simulink model "ASMCDUNG"  (R2022b)
settings: Solver=ode45  StartTime=0.0  StopTime=30  FixedStep=0.05  RelTol=1e-3
libraries: slpidlib x2
settings Model: Creator=vudin  LastModifiedBy=vudin
settings SolverCC: AlgebraicLoopSolver=TrustRegion
settings DataIOCC: ReturnWorkspaceOutputs=off
settings DebuggingCC: UnconnectedInputMsg=warning  UnconnectedOutputMsg=warning  UnconnectedLineMsg=warning  SFMachineParentedDataDiag=warning  ArithmeticOperatorsInVariantConditions=warning
settings ModelReferenceCC: EnableRefExpFcnMdlSchedulingChecks=on
settings SFSimCC: CustomCodeUndefinedFunction=UseInterfaceOnly

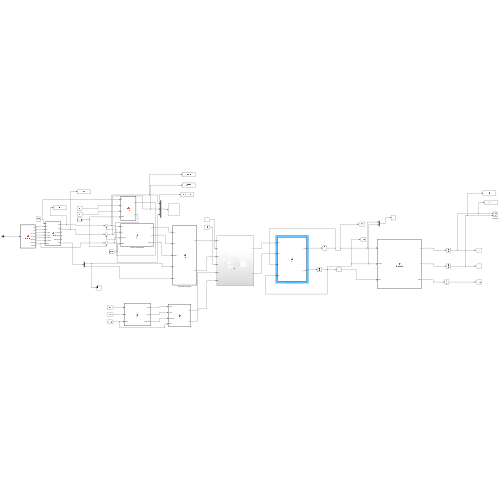
[thumbnail: Simulink's stored preview of the top-level diagram]
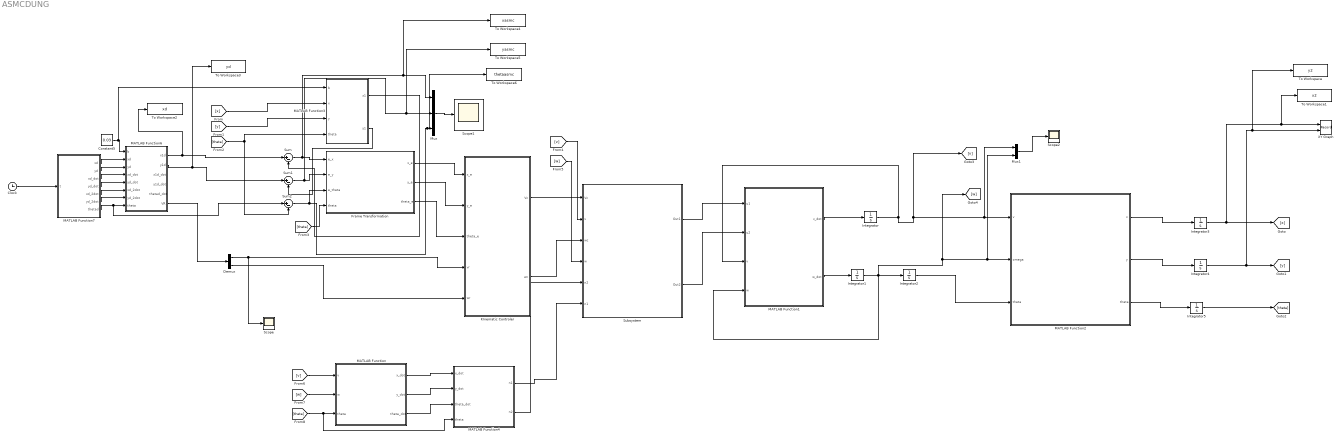
== system ASMCDUNG ==
  Clock : Clock
  Constant5 : Constant  Value=0.03
  Demux : Demux  Outputs=2
  Frame Transformation : MATLAB Function  TreatAsAtomicUnit=on
  Integrator{,1..5} (6 alike) : Integrator
  KInematic Controler : MATLAB Function  TreatAsAtomicUnit=on
  MATLAB Function : MATLAB Function  TreatAsAtomicUnit=on
  MATLAB Function1 : MATLAB Function  TreatAsAtomicUnit=on
  MATLAB Function2 : MATLAB Function  TreatAsAtomicUnit=on
  MATLAB Function3 : MATLAB Function  TreatAsAtomicUnit=on
  MATLAB Function4 : MATLAB Function  TreatAsAtomicUnit=on
  MATLAB Function6 : MATLAB Function  TreatAsAtomicUnit=on
  MATLAB Function7 : MATLAB Function  TreatAsAtomicUnit=on
  Mux : Mux  Inputs=3
  Mux1 : Mux  Inputs=2
  Scope : Scope
  Scope1 : Scope
  Scope2 : Scope
  Subsystem : Subsystem
  Sum : Sum  Inputs=|+-
  Sum1 : Sum  Inputs=|+-
  Sum2 : Sum  Inputs=|+-
  To Workspace : ToWorkspace  VariableName=y2  SampleTime=-1
  To Workspace1 : ToWorkspace  VariableName=x2  SampleTime=-1
  To Workspace2 : ToWorkspace  VariableName=xd  SaveFormat=Timeseries  SampleTime=-1
  To Workspace3 : ToWorkspace  VariableName=yd  SaveFormat=Timeseries  SampleTime=-1
  To Workspace4 : ToWorkspace  VariableName=xasmc  SaveFormat=Timeseries  SampleTime=-1
  To Workspace5 : ToWorkspace  VariableName=yasmc  SaveFormat=Timeseries  SampleTime=-1
  To Workspace6 : ToWorkspace  VariableName=thetaasmc  SaveFormat=Timeseries  SampleTime=-1
  XY Graph : Record  FileSettingsInternal="{\"entries\":[{\"content\":{\"excelSettings\":{\"content\":{},\"type\":\"Streamout.ExcelSettings\"}},\"type\":\"Streamout.FileSettingStorage\",\"uuid\":\"6435c98a-ca60-4c6a-9dec-2f97648765b9\"}],\"packageUris\":[\"http://schema.mathworks.com/mf0/streamout_blocks/R2020a\"],\"version\":\"1.0\"}"  Layout=[1 1]  SignalsInternal="{\"entries\":[{\"content\":{\"signals\":[{\"content\":{\"blockPath\":[\"ASMCDUNG/XY Graph\"],\"channel\":[],\"dimensions\":[1],\"domain\":\"ASMCDUNG/XY Graph\",\"lineColor\":\"#a2142f\",\"plots\":[1],\"port\":1,\"sid\":[\"\"],\"signalID\":19,\"signalName\":\"Integrator3\"},\"type\":\"RecordBlkView.Signal\",\"uuid\":\"5e08760f-4a30-4797-bcab-71919d67c0cf\"},{\"content\":{\"blockPath\":[\"ASMCDUNG/XY Graph\"],\"channel\":[],\"dimensions\":[1],\"domain\":\"ASMCDUNG/XY Graph\",\"lineColor\":\"#139fff\",\"plots\":[1],\"port\":2,\"sid\":[\"\"],\"signalID\":23,\"signalName\":\"Integrator4\"},\"type\":\"RecordBlkView.Signal\",\"uuid\":\"f2d516c6-4b6f-479c-badf-737930e26c05\"}]},\"type\":\"RecordBlkView.InputSignals\",\"uuid\":\"03edcad2-6278-41f4-8767-b85c0ff9a77c\"}],\"packageUris\":[\"http://schema.mathworks.com/mf0/streamout_blocks/R2020a\"],\"version\":\"1.0\"}"  VisualizationBindings="{\"xyplotplugin\":{\"info\":[{\"series\":[{\"bindingParametersList\":[{\"parameter\":\"X-Axis\",\"signalID\":19,\"signalName\":\"Integrator3\"},{\"parameter\":\"Y-Axis\",\"signalID\":23,\"signalName\":\"Integrator4\"}],\"seriesID\":10262}],\"subplotID\":1}]}}"  CompatibilityTag=XY  st=-1
  wires:
  Frame Transformation/2(y_e) -> KInematic Controler/2(y_e)
  MATLAB Function3/1(x1) -> Sum/2
  Integrator4/1 -> To Workspace/1, XY Graph/2, [y]
  [theta] -> Frame Transformation/4(theta)
  [theta] -> MATLAB Function4/4(theta), MATLAB Function/3(theta)
  MATLAB Function/2(y_dot) -> MATLAB Function4/2(y_dot)
  [w] -> MATLAB Function/2(w)
  Subsystem/2(Out2) -> MATLAB Function1/2(u2)
  [x] -> MATLAB Function3/2(x)
  Demux/2 -> KInematic Controler/5(wr)
  [v] -> MATLAB Function/1(v)
  MATLAB Function7/4(yd_dot) -> MATLAB Function6/5(yd_dot)
  Frame Transformation/1(x_e) -> KInematic Controler/1(x_e)
  [y] -> MATLAB Function3/3(y)
  Frame Transformation/3(theta_e) -> KInematic Controler/3(theta_e)
  MATLAB Function/3(theta_dot) -> MATLAB Function4/3(theta_dot)
  Sum1/1 -> To Workspace5/1, Mux/2, Frame Transformation/2(e_y)
  Sum2/1 -> To Workspace6/1, Mux/3, Frame Transformation/3(e_theta)
  MATLAB Function7/6(yd_2dot) -> MATLAB Function6/7(yd_2dot)
  Demux/1 -> Scope/1, KInematic Controler/4(vr)
  [v] -> Subsystem/2(v)
  Subsystem/1(Out1) -> MATLAB Function1/1(u1)
  MATLAB Function7/1(xd) -> MATLAB Function6/2(xd)
  MATLAB Function2/1(x) -> Integrator3/1
  Mux1/1 -> Scope2/1
  MATLAB Function7/7(thetad) -> Sum2/1, MATLAB Function6/8(theta)
  KInematic Controler/2(wc) -> Subsystem/3(wc)
  Constant5/1 -> MATLAB Function3/1(b), MATLAB Function6/1(b)
  MATLAB Function7/2(yd) -> MATLAB Function6/3(yd)
  MATLAB Function7/3(xd_dot) -> MATLAB Function6/4(xd_dot)
  MATLAB Function6/6(VR) -> Demux/1
  Sum/1 -> Frame Transformation/1(e_x), To Workspace4/1, Mux/1
  Integrator/1 -> MATLAB Function1/3(v), [v], Mux1/1, MATLAB Function2/1(v)
  MATLAB Function3/2(y1) -> Sum1/2
  Integrator5/1 -> [theta]
  [w] -> Subsystem/4(w)
  MATLAB Function4/2(n2) -> Subsystem/5(n2)
  MATLAB Function1/1(v_dot) -> Integrator/1
  MATLAB Function1/2(w_dot) -> Integrator1/1
  MATLAB Function6/1(x1d) -> To Workspace2/1, Sum/1
  MATLAB Function/1(x_dot) -> MATLAB Function4/1(x_dot)
  MATLAB Function2/2(y) -> Integrator4/1
  MATLAB Function6/2(y1d) -> To Workspace3/1, Sum1/1
  MATLAB Function2/3(theta) -> Integrator5/1
  [theta] -> Sum2/2, MATLAB Function3/4(theta)
  Integrator3/1 -> To Workspace1/1, XY Graph/1, [x]
  KInematic Controler/1(Vc) -> Subsystem/1(Vc)
  Integrator1/1 -> [w], Mux1/2, MATLAB Function2/2(omega), MATLAB Function1/4(w), Integrator2/1
  MATLAB Function4/1(n1) -> Subsystem/6(n1)
  Mux/1 -> Scope1/1
  Integrator2/1 -> MATLAB Function2/3("theta ")
  MATLAB Function7/5(xd_2dot) -> MATLAB Function6/6(xd_2dot)
  Clock/1 -> MATLAB Function7/1(t)

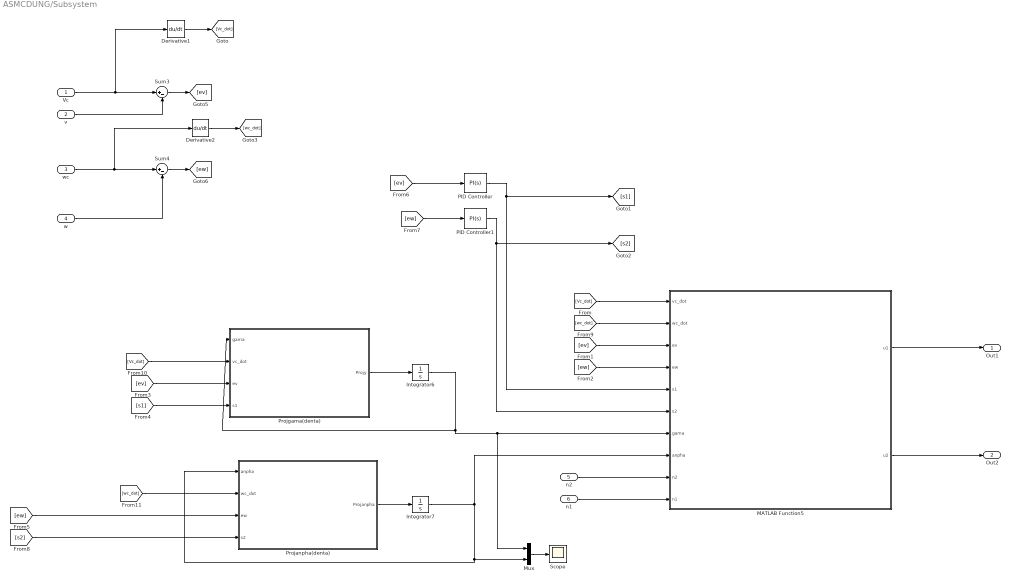
== system ASMCDUNG/Subsystem ==
  Vc : Inport
  v : Inport  Port=2
  wc : Inport  Port=3
  w : Inport  Port=4
  n2 : Inport  Port=5
  n1 : Inport  Port=6
  Derivative1 : Derivative
  Derivative2 : Derivative
  Integrator6 : Integrator
  Integrator7 : Integrator
  MATLAB Function5 : MATLAB Function  TreatAsAtomicUnit=on
  Mux : Mux  Inputs=2
  PID Controller : slpidlib/PID Controller  Controller=PI  Form=Parallel  TimeDomain=Continuous-time  UseExternalTs=off  SampleTime=-1  IntegratorMethod=Forward Euler  FilterMethod=Forward Euler  ControllerParametersSource=internal  P=3.4  I=1  UseKiTs=off  D=0  N=100  UseFilter=on  TunerSelectOption=Transfer Function Based (PID Tuner App)  InitialConditionSource=internal  InitialConditionForIntegrator=0  InitialConditionForFilter=0  DifferentiatorICPrevScaledInput=0  ExternalReset=none  TrackingMode=off  Kt=1  LimitOutput=off  SatLimitsSource=internal  UpperSaturationLimit=inf  LowerSaturationLimit=-inf  LinearizeAsGain=on  AntiWindupMode=none  Kb=1  LimitIntegrator=off  UpperIntegratorSaturationLimit=inf  LowerIntegratorSaturationLimit=-inf  POutMin=[]  POutMax=[]  IOutMin=[]  IOutMax=[]  DOutMin=[]  DOutMax=[]  NOutMin=[]  NOutMax=[]  SumOutMin=[]  SumOutMax=[]  SaturationOutMin=[]  SaturationOutMax=[]  PParamMin=[]  PParamMax=[]  IParamMin=[]  IParamMax=[]  DParamMin=[]  DParamMax=[]  NParamMin=[]  NParamMax=[]  KbParamMin=[]  KbParamMax=[]  KtParamMin=[]  KtParamMax=[]  KbOutMin=[]  KbOutMax=[]  KtOutMin=[]  KtOutMax=[]  IntegratorOutMin=[]  IntegratorOutMax=[]  FilterOutMin=[]  FilterOutMax=[]  SumI1OutMin=[]  SumI1OutMax=[]  SumI2OutMin=[]  SumI2OutMax=[]  SumI3OutMin=[]  SumI3OutMax=[]  SumI4OutMin=[]  SumI4OutMax=[]  SumDOutMin=[]  SumDOutMax=[]  DifferentiatorOutMin=[]  DifferentiatorOutMax=[]  FilterDiffOutCoefMin=[]  FilterDiffOutCoefMax=[]  ReciprocalOutMin=[]  ReciprocalOutMax=[]  SumDenOutMin=[]  SumDenOutMax=[]  SumNumOutMin=[]  SumNumOutMax=[]  DivideOutMin=[]  DivideOutMax=[]  UdiffTsProdOutMin=[]  UdiffTsProdOutMax=[]  NTsProdOutMin=[]  NTsProdOutMax=[]  UintegralTsProdOutMin=[]  UintegralTsProdOutMax=[]  UngainTsProdOutMin=[]  UngainTsProdOutMax=[]  ClampingZeroOutDataTypeStr=Inherit: Inherit via back propagation  ClampingZeroOutMin=[]  ClampingZeroOutMax=[]  FilterDenConstantOutDataTypeStr=Inherit: Inherit via back propagation  FilterDenConstantOutMin=[]  FilterDenConstantOutMax=[]  PCopyOutDataTypeStr=Inherit: Inherit via back propagation  PCopyOutMin=[]  PCopyOutMax=[]  NCopyOutDataTypeStr=Inherit: Inherit via back propagation  NCopyOutMin=[]  NCopyOutMax=[]  IntegratorContinuousStateAttributes=''  IntegratorStateMustResolveToSignalObject=off  IntegratorRTWStateStorageClass=Auto  FilterContinuousStateAttributes=''  FilterStateMustResolveToSignalObject=off  FilterRTWStateStorageClass=Auto  ParallelPVariant=InternalParameters  IdealPVariant=Disabled  IVariant=InternalParameters  DVariant=Disabled  IntegratorVariant=Continuous  SatVariant=Disabled  AWVariant=Passthrough  PCopyVariant=Disabled  TRVariant=Disabled  FdbkBlocksVariant=Forward  IdealPFdbkVariant=Disabled  SatFdbkVariant=Disabled  DerivativeFilterVariant=Disabled  NVariant=Disabled  NCopyVariant=Disabled_SignalSpec  FilterICVariant=Disabled  IntegratorICVariant=InternalICs  ExternalResetVariant=Disabled  TRSumVariant=Passthrough  SumFdbkVariant=Disabled  SumVariant=Sum_PI  TsampFilterVariant=InternalTs  TsampNgainVariant=Passthrough  TsampIntegralVariant=Passthrough  ExternalSaturationOutDataTypeStr=Inherit: Same as second input
  PID Controller1 : slpidlib/PID Controller  Controller=PI  Form=Parallel  TimeDomain=Continuous-time  UseExternalTs=off  SampleTime=-1  IntegratorMethod=Forward Euler  FilterMethod=Forward Euler  ControllerParametersSource=internal  P=4  I=2  UseKiTs=off  D=0  N=100  UseFilter=on  TunerSelectOption=Transfer Function Based (PID Tuner App)  InitialConditionSource=internal  InitialConditionForIntegrator=0  InitialConditionForFilter=0  DifferentiatorICPrevScaledInput=0  ExternalReset=none  TrackingMode=off  Kt=1  LimitOutput=off  SatLimitsSource=internal  UpperSaturationLimit=inf  LowerSaturationLimit=-inf  LinearizeAsGain=on  AntiWindupMode=none  Kb=1  LimitIntegrator=off  UpperIntegratorSaturationLimit=inf  LowerIntegratorSaturationLimit=-inf  POutMin=[]  POutMax=[]  IOutMin=[]  IOutMax=[]  DOutMin=[]  DOutMax=[]  NOutMin=[]  NOutMax=[]  SumOutMin=[]  SumOutMax=[]  SaturationOutMin=[]  SaturationOutMax=[]  PParamMin=[]  PParamMax=[]  IParamMin=[]  IParamMax=[]  DParamMin=[]  DParamMax=[]  NParamMin=[]  NParamMax=[]  KbParamMin=[]  KbParamMax=[]  KtParamMin=[]  KtParamMax=[]  KbOutMin=[]  KbOutMax=[]  KtOutMin=[]  KtOutMax=[]  IntegratorOutMin=[]  IntegratorOutMax=[]  FilterOutMin=[]  FilterOutMax=[]  SumI1OutMin=[]  SumI1OutMax=[]  SumI2OutMin=[]  SumI2OutMax=[]  SumI3OutMin=[]  SumI3OutMax=[]  SumI4OutMin=[]  SumI4OutMax=[]  SumDOutMin=[]  SumDOutMax=[]  DifferentiatorOutMin=[]  DifferentiatorOutMax=[]  FilterDiffOutCoefMin=[]  FilterDiffOutCoefMax=[]  ReciprocalOutMin=[]  ReciprocalOutMax=[]  SumDenOutMin=[]  SumDenOutMax=[]  SumNumOutMin=[]  SumNumOutMax=[]  DivideOutMin=[]  DivideOutMax=[]  UdiffTsProdOutMin=[]  UdiffTsProdOutMax=[]  NTsProdOutMin=[]  NTsProdOutMax=[]  UintegralTsProdOutMin=[]  UintegralTsProdOutMax=[]  UngainTsProdOutMin=[]  UngainTsProdOutMax=[]  ClampingZeroOutDataTypeStr=Inherit: Inherit via back propagation  ClampingZeroOutMin=[]  ClampingZeroOutMax=[]  FilterDenConstantOutDataTypeStr=Inherit: Inherit via back propagation  FilterDenConstantOutMin=[]  FilterDenConstantOutMax=[]  PCopyOutDataTypeStr=Inherit: Inherit via back propagation  PCopyOutMin=[]  PCopyOutMax=[]  NCopyOutDataTypeStr=Inherit: Inherit via back propagation  NCopyOutMin=[]  NCopyOutMax=[]  IntegratorContinuousStateAttributes=''  IntegratorStateMustResolveToSignalObject=off  IntegratorRTWStateStorageClass=Auto  FilterContinuousStateAttributes=''  FilterStateMustResolveToSignalObject=off  FilterRTWStateStorageClass=Auto  ParallelPVariant=InternalParameters  IdealPVariant=Disabled  IVariant=InternalParameters  DVariant=Disabled  IntegratorVariant=Continuous  SatVariant=Disabled  AWVariant=Passthrough  PCopyVariant=Disabled  TRVariant=Disabled  FdbkBlocksVariant=Forward  IdealPFdbkVariant=Disabled  SatFdbkVariant=Disabled  DerivativeFilterVariant=Disabled  NVariant=Disabled  NCopyVariant=Disabled_SignalSpec  FilterICVariant=Disabled  IntegratorICVariant=InternalICs  ExternalResetVariant=Disabled  TRSumVariant=Passthrough  SumFdbkVariant=Disabled  SumVariant=Sum_PI  TsampFilterVariant=InternalTs  TsampNgainVariant=Passthrough  TsampIntegralVariant=Passthrough  ExternalSaturationOutDataTypeStr=Inherit: Same as second input
  Projanpha(denta) : MATLAB Function  TreatAsAtomicUnit=on
  Projgama(denta) : MATLAB Function  TreatAsAtomicUnit=on
  Scope : Scope
  Sum3 : Sum  Inputs=|+-
  Sum4 : Sum  Inputs=|+-
  Out1 : Outport  VectorParamsAs1DForOutWhenUnconnected=off
  Out2 : Outport  Port=2  VectorParamsAs1DForOutWhenUnconnected=off
  wires:
  Vc/1 -> Derivative1/1, Sum3/1
  [ev] -> PID Controller/1
  Sum3/1 -> [ev]
  [ew] -> PID Controller1/1
  Sum4/1 -> [ew]
  v/1 -> Sum3/2
  w/1 -> Sum4/2
  wc/1 -> Derivative2/1, Sum4/1
  MATLAB Function5/1(u1) -> Out1/1
  MATLAB Function5/2(u2) -> Out2/1
  Projgama(denta)/1(Projy) -> Integrator6/1
  Integrator7/1 -> Mux/2, Projanpha(denta)/1(anpha), MATLAB Function5/8(anpha)
  Projanpha(denta)/1(Projanpha) -> Integrator7/1
  Integrator6/1 -> Projgama(denta)/1(gama), Mux/1, MATLAB Function5/7(gama)
  [ev] -> MATLAB Function5/3(ev)
  [ew] -> MATLAB Function5/4(ew)
  PID Controller/1 -> [s1], MATLAB Function5/5(s1)
  PID Controller1/1 -> MATLAB Function5/6(s2), [s2]
  [ev] -> Projgama(denta)/3(ev)
  [s1] -> Projgama(denta)/4(s1)
  [ew] -> Projanpha(denta)/3(ew)
  [s2] -> Projanpha(denta)/4(s2)
  n1/1 -> MATLAB Function5/10(n1)
  n2/1 -> MATLAB Function5/9(n2)
  Derivative1/1 -> [Vc_dot]
  Derivative2/1 -> [wc_dot]
  [wc_dot] -> MATLAB Function5/2(wc_dot)
  [Vc_dot] -> MATLAB Function5/1(vc_dot)
  [Vc_dot] -> Projgama(denta)/2(vc_dot)
  [wc_dot] -> Projanpha(denta)/2(wc_dot)
  Mux/1 -> Scope/1

== matlab function ASMCDUNG/MATLAB Function ==
  data: x_dot output; y_dot output; v input; w input; theta input; theta_dot output
function [x_dot,y_dot,theta_dot] = fcn(v,w,theta)

S=[cos(theta) 0;
 sin(theta) 0;
 0 1];
ve=[v;w];
q=S*ve;
x_dot=q(1);

y_dot=q(2);
theta_dot=q(3);

== matlab function ASMCDUNG/MATLAB Function4 ==
  data: x_dot input; n1 output; y_dot input; theta_dot input; n2 output; theta input
function [n1,n2]= fcn(x_dot,y_dot,theta_dot,theta)

R=0.076;
L=0.02;
C=[x_dot;y_dot;theta_dot];

D=[R*cos(theta)/2 R*cos(theta)/2;R*sin(theta)/2 R*sin(theta)/2;R/(2*L) R/(2*L)];

E=D\C;

n1=E(1);
n2=E(2);

== matlab function ASMCDUNG/MATLAB Function7 ==
  data: t input; xd output; yd output; xd_dot output; yd_dot output; xd_2dot output; yd_2dot output; thetad output
function [xd,yd,xd_dot,yd_dot,xd_2dot,yd_2dot,thetad] = quydao(t)
%% Khoi tao quy dao chuyen dong
R=5; %ban kinh quy dao
w=0.2; %rad/s =2*pi*f f=w/2/pi -> T=1/f
xd=R*cos(w*t);
yd=R*sin(w*t);
xd_dot=-R*w*sin(w*t);
yd_dot=R*w*cos(w*t);
x0d_dot=-R*w*sin(w);
y0d_dot=R*w*cos(w);
xd_2dot=-R*w^2*cos(w*t);
yd_2dot=-R*w^2*sin(w*t);
theta0=atan2(y0d_dot,x0d_dot)-w;
thetad=w*t + theta0;

== matlab function ASMCDUNG/Subsystem/MATLAB Function5 ==
  data: vc_dot input; u1 output; wc_dot input; ev input; ew input; u2 output; s1 input; s2 input; gama input; anpha input; n2 input; n1 input
function [u1,u2] = fcn(vc_dot,wc_dot,ev,ew,s1,s2,gama,anpha,n2,n1)
R=0.095;%bánh kính bánh xe
L=0.24; %khoảng cách từ tâm bánh đến tâm DDMR
Iw=0.0023; %momen quán tính của bánh xe dẫn động với bộ truyền động quanh trục bánh xe
mc=17; %khối lượng khi không có bánh và bộ truyền động
mw=0.5; %khối lượng mỗi bánh bao gồm cả hệ truyền động
d=0.05; %khoảng cách giữa điểm gốc và khối tâm
Ic=0.537; %momen quán tính của robot với trục xr đi qua tâm
Im=0.0011; %momen quán tính mỗi bánh dẫn động 

m=mc + 2*mw;
I= Ic+ mc*d^2 +2*mw*L^2 +2*Im;
m0= m + (2*Iw)/R^2;
i0= I + (2*L^2*Iw)/R^2;

beta=0.5;
e=0.05;
K1=1000;
K2=1200;

u1=gama*(vc_dot + beta*ev)+K1*s1 + n1*tanh(s1/e);
u2=anpha*(wc_dot + beta*ew)+ K2*s2+ n2*tanh(s2/e);

== matlab function ASMCDUNG/Subsystem/Projanpha(denta) ==
  data: anpha input; Projanpha output; wc_dot input; ew input; s2 input
function Projanpha  = fcn(anpha,wc_dot,ew,s2)

R=0.095;%bánh kính bánh xe
L=0.24; %khoảng cách từ tâm bánh đến tâm DDMR
Iw=0.0023; %momen quán tính của bánh xe dẫn động với bộ truyền động quanh trục bánh xe
mc=17; %khối lượng khi không có bánh và bộ truyền động
mw=0.5; %khối lượng mỗi bánh bao gồm cả hệ truyền động
d=0.05; %khoảng cách giữa điểm gốc và khối tâm
Ic=0.537; %momen quán tính của robot với trục xr đi qua tâm
Im=0.0011; %momen quán tính mỗi bánh dẫn động 

m=mc + 2*mw;
I= Ic+ mc*d^2 +2*mw*L^2 +2*Im;
m0= m + (2*Iw)/R^2;
i0= I + (2*L^2*Iw)/R^2;

beta=0.5;
b=0.5;
denta2=-b*s2*(wc_dot + beta*ew);
anphamax=i0*R/L;
anphamin=i0*R/L;
if anpha==anphamax && denta2>0
  Projanpha=0;
elseif anpha==anphamin && denta2<0
   Projanpha=0;
else
    Projanpha=denta2;
end
end

== matlab function ASMCDUNG/Subsystem/Projgama(denta) ==
  data: gama input; Projy output; vc_dot input; ev input; s1 input
function Projy  = fcn(gama,vc_dot,ev,s1)
R=0.095;%bánh kính bánh xe
L=0.24; %khoảng cách từ tâm bánh đến tâm DDMR
Iw=0.0023; %momen quán tính của bánh xe dẫn động với bộ truyền động quanh trục bánh xe
mc=17; %khối lượng khi không có bánh và bộ truyền động
mw=0.5; %khối lượng mỗi bánh bao gồm cả hệ truyền động
d=0.05; %khoảng cách giữa điểm gốc và khối tâm
Ic=0.537; %momen quán tính của robot với trục xr đi qua tâm
Im=0.0011; %momen quán tính mỗi bánh dẫn động 

m=mc + 2*mw;
I= Ic+ mc*d^2 +2*mw*L^2 +2*Im;
m0= m + (2*Iw)/R^2;
i0= I + (2*L^2*Iw)/R^2;



beta=0.5;
a=0.5;
denta=-a*s1*(vc_dot + beta*ev);
gamamax=m0*R;
gamamin=-m0*R;
if gama==gamamax && denta>0
  Projy=0;
elseif gama==gamamin && denta<0
   Projy=0;
else
    Projy=denta;
end
end

== matlab function ASMCDUNG/Frame Transformation ==
  data: e_x input; x_e output; e_y input; e_theta input; y_e output; theta_e output; theta input
function [x_e,y_e,theta_e] = fcn(e_x,e_y,e_theta,theta)
A=[cos(theta) sin(theta) 0;-sin(theta) cos(theta) 0;0 0 1];
B=[e_x;e_y;e_theta];
C=A*B;
x_e=C(1);
y_e=C(2);
theta_e=C(3);
% công thức 45

== matlab function ASMCDUNG/KInematic Controler ==
  data: x_e input; Vc output; y_e input; theta_e input; wc output; vr input; wr input
function [Vc,wc] = fcn(x_e,y_e,theta_e,vr,wr)
Vc=vr*cos(theta_e)+ x_e;
wc=wr+vr*(y_e + sin(theta_e));

%công thức 46

== matlab function ASMCDUNG/MATLAB Function3 ==
  data: b input; x1 output; y1 output; x input; y input; theta input
function [x1,y1] = quydao(b,x,y,theta)
%% Thiet lap quy dao chuyen dong cho robot
%theta=atan2(yd_dot,xd_dot);
x1=x+b*cos(theta);
y1=y+b*sin(theta);

== matlab function ASMCDUNG/MATLAB Function1 ==
  data: u1 input; v_dot output; u2 input; v input; w input; w_dot output
function [v_dot,w_dot]=fcn(u1,u2,v,w)
R=0.095;%bánh kính bánh xe
L=0.24; %khoảng cách từ tâm bánh đến tâm DDMR
Iw=0.0023; %momen quán tính của bánh xe dẫn động với bộ truyền động quanh trục bánh xe
mc=17; %khối lượng khi không có bánh và bộ truyền động
mw=0.5; %khối lượng mỗi bánh bao gồm cả hệ truyền động
d=0.05; %khoảng cách giữa điểm gốc và khối tâm
Ic=0.537; %momen quán tính của robot với trục xr đi qua tâm
Im=0.0011; %momen quán tính mỗi bánh dẫn động 

m=mc + 2*mw;
I= Ic+ mc*d^2 +2*mw*L^2 +2*Im;
m0= m + (2*Iw)/R^2;
i0= I + (2*L^2*Iw)/R^2;

M=[m0 0;0 i0];
V=[0 -mc*d*w;mc*d*w 0];
T=[1/R 0;0 L/R];
u=[u1;u2];
k=[v;w];

N=T*u-V*k;
Z=inv(M)*N;
v_dot=Z(1);
w_dot=Z(2);

== matlab function ASMCDUNG/MATLAB Function2 ==
  data: v input; x output; omega input; theta input; y output; theta output
function [x,y,theta]=Kinematics(v,omega,theta)

S=[cos(theta) 0;
 sin(theta) 0;
 0 1];
ve=[v;omega];
qdot=S*ve;
x=qdot(1);

y=qdot(2);
theta=qdot(3);

== matlab function ASMCDUNG/MATLAB Function6 ==
  data: b input; x1d output; y1d output; x1d_dot output; y1d_dot output; thetad_dot output; xd input; yd input; xd_dot input; yd_dot input; xd_2dot input; yd_2dot input; theta input; VR output
function [x1d,y1d,x1d_dot,y1d_dot,thetad_dot,VR] = quydao(b,xd,yd,xd_dot,yd_dot,xd_2dot,yd_2dot,theta)
%% Thiet lap quy dao chuyen dong cho robot
%theta=atan2(yd_dot,xd_dot);
x1d=xd+b*cos(theta);
y1d=yd+b*sin(theta);
wd=(yd_2dot*xd_dot - xd_2dot*yd_dot)/(xd_dot^2+yd_dot^2);
x1d_dot=xd_dot-b*wd*sin(theta);
y1d_dot=yd_dot+b*wd*cos(theta);
thetad_dot=wd;
rot=[cos(theta) 0; sin(theta) 0; 0 1];
p_dot=[xd_dot; yd_dot; wd];
VR=rot\p_dot;
